simulink model "RCAM_simulation"  (R2024a)
settings: Solver=VariableStepAuto  StartTime=0.0  StopTime=t_final  RelTol=1e-3
values from neighbouring files (symbols this model uses):
  x0 = [85 ... (first row only)    [RCAM_initialConds.m]    (also in RCAM_run.m)
undefined symbols (not defined in the file or in its folder): RCAM_dynamics
settings Model: Creator=jake0  LastModifiedBy=jake0

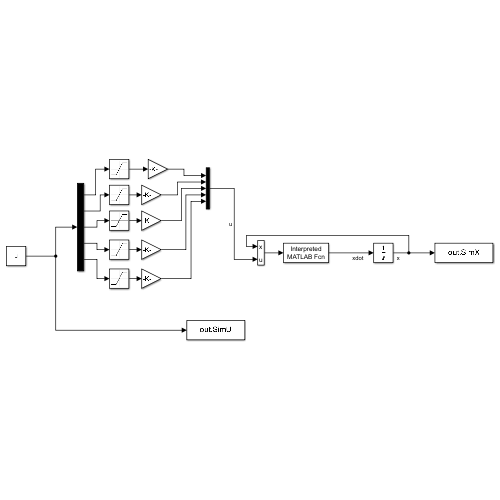
[thumbnail: Simulink's stored preview of the top-level diagram]
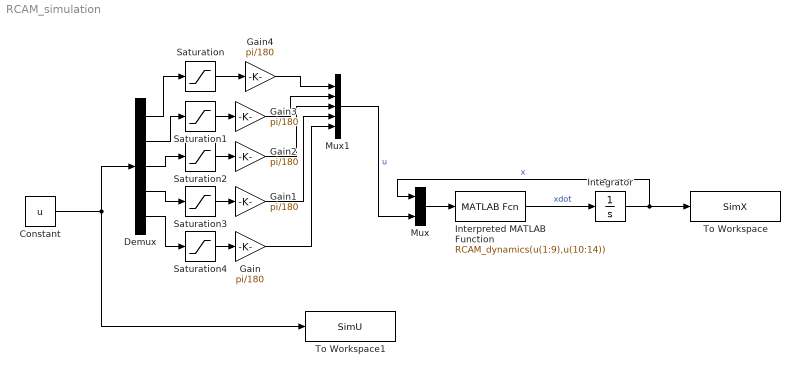
== system RCAM_simulation ==
  Constant : Constant  Value=u
  Demux : Demux  Outputs=5
  Gain{,1..4} (5 alike) : Gain  Gain=pi/180
  Integrator : Integrator  InitialCondition=x0
  Interpreted MATLAB Function : MATLABFcn  MATLABFcn=RCAM_dynamics(u(1:9),u(10:14))
  Mux : Mux  Inputs=2
      settings: DisplayOption=signals
  Mux1 : Mux  Inputs=5
  Saturation : Saturate  UpperLimit=25*pi/180  LowerLimit=-25*pi/180
  Saturation1 : Saturate  UpperLimit=10*pi/180  LowerLimit=-25*pi/180
  Saturation2 : Saturate  UpperLimit=30*pi/180  LowerLimit=-30*pi/180
  Saturation3 : Saturate  UpperLimit=10*pi/180  LowerLimit=0.5*pi/180
  Saturation4 : Saturate  UpperLimit=10*pi/180  LowerLimit=0.5*pi/180
  To Workspace : ToWorkspace  VariableName=SimX  SaveFormat=Timeseries  SampleTime=-1
  To Workspace1 : ToWorkspace  VariableName=SimU  SaveFormat=Timeseries  SampleTime=-1
  wires:
  Integrator/1 -> Mux/1, To Workspace/1  "x"
  Interpreted MATLAB Function/1 -> Integrator/1  "xdot"
  Constant/1 -> Demux/1, To Workspace1/1
  Mux/1 -> Interpreted MATLAB Function/1
  Demux/1 -> Saturation/1
  Demux/2 -> Saturation1/1
  Demux/3 -> Saturation2/1
  Demux/4 -> Saturation3/1
  Demux/5 -> Saturation4/1
  Saturation4/1 -> Gain/1
  Saturation3/1 -> Gain1/1
  Saturation1/1 -> Gain3/1
  Saturation2/1 -> Gain2/1
  Saturation/1 -> Gain4/1
  Gain4/1 -> Mux1/1
  Gain3/1 -> Mux1/2
  Gain2/1 -> Mux1/3
  Gain1/1 -> Mux1/4
  Gain/1 -> Mux1/5
  Mux1/1 -> Mux/2  "u"
